simulink model "actuators"  (R2024a)
settings: configuration reference "standardSILConfiguraitonParams" (kept outside this file)
undefined symbols (not defined in the file): aileronDeflRateLimit_degps, elevatorDeflRateLimit_degps, maxAilDefl_deg, maxElevatorDefl_deg, maxRudderDefl_deg, rudderDeflRateLimit_degps, ServosF16Bus, tauAilerons_s, tauElevator_s, tauRudder_s
settings Model: Creator=GTAR  LastModifiedBy=jerem
settings ConfigSetRef: SourceName=standardSILConfiguraitonParams  SourceLocation=Base Workspace

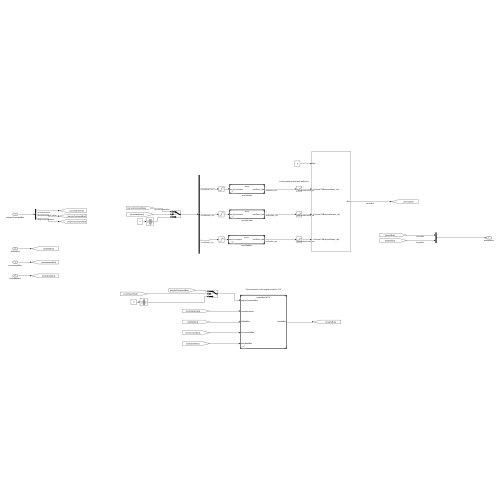
[thumbnail: Simulink's stored preview of the top-level diagram]
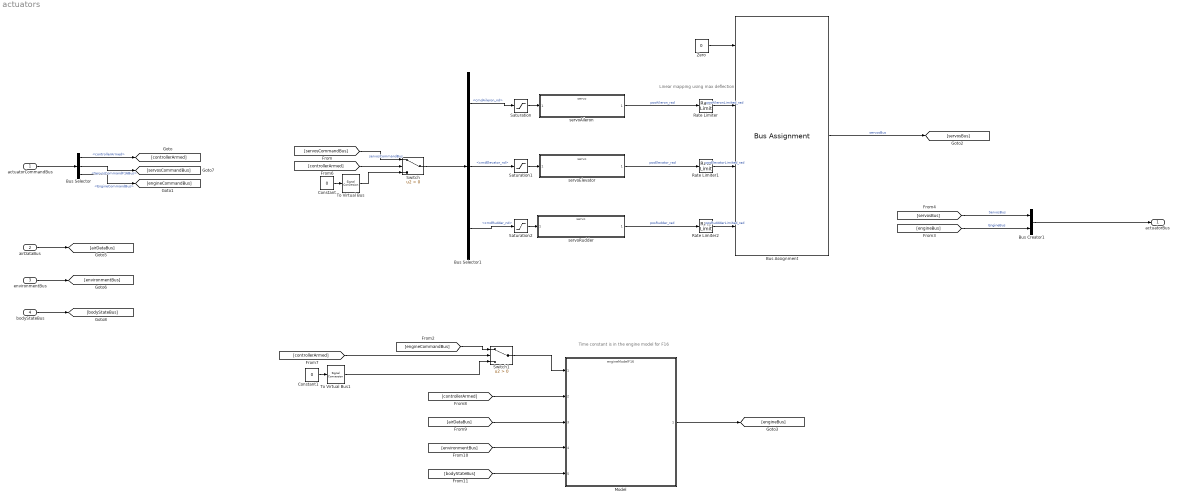
== system actuators ==
  note: Linear mapping using max deflection
  note: Time constant is in the engine model for F16
  actuatorCommandBus : Inport  OutDataTypeStr=Bus: ActuatorCommandBus
  airDataBus : Inport  Port=2  OutDataTypeStr=Bus: AirData
  environmentBus : Inport  Port=3  OutDataTypeStr=Bus: EnvironmentBus
  bodyStateBus : Inport  Port=4  OutDataTypeStr=Bus: BodyStateBus
  Bus Assignment : BusAssignment  AssignedSignals=ServosF16Bus.posAileron_rad,ServosF16Bus.posElevator_rad,ServosF16Bus.posRudder_rad
  Bus Creator1 : BusCreator  Inputs=2  OutDataTypeStr=Bus: ActuatorBus
  Bus Selector : BusSelector  OutputSignals=controllerArmed,ServosCommandBus.ServosCommandF16Bus,EngineCommandBus
  Bus Selector1 : BusSelector  OutputSignals=cmdAileron_nd,cmdElevator_nd,cmdRudder_nd
  Constant : Constant  Value=0  VectorParams1D=off  OutDataTypeStr=Bus: ServosCommandF16Bus  SampleTime=-1
  Constant1 : Constant  Value=0  OutDataTypeStr=Bus: EngineCommandBus
  Model : ModelReference  ModelNameDialog=engineModelF16.slx  SimulationMode=Normal  ModelReferenceVersion=1.109
  Rate Limiter : RateLimiter  RisingSlewLimit=deg2rad(aileronDeflRateLimit_degps)  FallingSlewLimit=-deg2rad(aileronDeflRateLimit_degps)  SampleTimeMode=inherited
  Rate Limiter1 : RateLimiter  RisingSlewLimit=deg2rad(elevatorDeflRateLimit_degps)  FallingSlewLimit=-deg2rad(elevatorDeflRateLimit_degps)  SampleTimeMode=inherited
  Rate Limiter2 : RateLimiter  RisingSlewLimit=deg2rad(rudderDeflRateLimit_degps)  FallingSlewLimit=deg2rad(-rudderDeflRateLimit_degps)  SampleTimeMode=inherited
  Saturation : Saturate  UpperLimit=1  LowerLimit=-1
  Saturation1 : Saturate  UpperLimit=1  LowerLimit=-1
  Saturation2 : Saturate  UpperLimit=1  LowerLimit=-1
  Switch : Switch  Criteria=u2 > Threshold  SaturateOnIntegerOverflow=off  InputSameDT=off
  Switch1 : Switch  Criteria=u2 > Threshold  SaturateOnIntegerOverflow=off  InputSameDT=off
  To Virtual Bus : SignalConversion  ConversionOutput=Virtual bus  OverrideOpt=off
  To Virtual Bus1 : SignalConversion  ConversionOutput=Virtual bus  OverrideOpt=off
  Zero : Constant  Value=0  OutDataTypeStr=Bus: ServosBus
  servoAileron : ModelReference  ModelNameDialog=servo.slx  UsingDefaultArgumentValue=0,0,0  SimulationMode=Normal  ModelReferenceVersion=1.21  scale=deg2rad(maxAilDefl_deg)  tfNumerator=1  tfDenominator=[tauAilerons_s 1]
  servoElevator : ModelReference  ModelNameDialog=servo.slx  UsingDefaultArgumentValue=0,0,0  SimulationMode=Normal  ModelReferenceVersion=1.21  scale=deg2rad(maxElevatorDefl_deg)  tfNumerator=1  tfDenominator=[tauElevator_s 1]
  servoRudder : ModelReference  ModelNameDialog=servo.slx  UsingDefaultArgumentValue=0,0,0  SimulationMode=Normal  ModelReferenceVersion=1.21  scale=deg2rad(maxRudderDefl_deg)  tfNumerator=1  tfDenominator=[tauRudder_s 1]
  actuatorBus : Outport  OutDataTypeStr=Bus: ActuatorBus
  wires:
  Bus Assignment/1 -> [servosBus]  "servosBus"
  Model/1 -> [engineBus]
  [engineBus] -> Bus Creator1/2  "EngineBus"
  [servosBus] -> Bus Creator1/1  "ServosBus"
  Bus Selector1/1 -> Saturation/1  "<cmdAileron_nd>"
  Bus Selector1/2 -> Saturation1/1  "<cmdElevator_nd>"
  Bus Selector1/3 -> Saturation2/1  "<cmdRudder_nd>"
  Bus Creator1/1 -> actuatorBus/1
  [servosCommandBus] -> Switch/1  "servosCommandBus"
  Switch/1 -> Bus Selector1/1
  [controllerArmed] -> Switch/2
  Constant/1 -> To Virtual Bus/1
  Switch1/1 -> Model/1
  Constant1/1 -> To Virtual Bus1/1
  [controllerArmed] -> Switch1/2
  To Virtual Bus/1 -> Switch/3
  To Virtual Bus1/1 -> Switch1/3
  airDataBus/1 -> [airDataBus]
  [airDataBus] -> Model/3
  environmentBus/1 -> [environmentBus]
  [environmentBus] -> Model/4
  bodyStateBus/1 -> [bodyStateBus]
  [bodyStateBus] -> Model/5
  [controllerArmed] -> Model/2
  actuatorCommandBus/1 -> Bus Selector/1
  Bus Selector/1 -> [controllerArmed]  "<controllerArmed>"
  Bus Selector/2 -> [servosCommandBus]  "<ServosCommandF16Bus>"
  Bus Selector/3 -> [engineCommandBus]  "<EngineCommandBus>"
  Zero/1 -> Bus Assignment/1
  servoElevator/1 -> Rate Limiter1/1  "posElevator_rad"
  servoRudder/1 -> Rate Limiter2/1  "posRudder_rad"
  servoAileron/1 -> Rate Limiter/1  "posAileron_rad"
  [engineCommandBus] -> Switch1/1
  Rate Limiter/1 -> Bus Assignment/2  "posAileronLimited_rad"
  Rate Limiter1/1 -> Bus Assignment/3  "posElevatorLimited_rad"
  Rate Limiter2/1 -> Bus Assignment/4  "posRuddderLimited_rad"
  Saturation2/1 -> servoRudder/1
  Saturation1/1 -> servoElevator/1
  Saturation/1 -> servoAileron/1
